simulink model "ModeSelectionRing"  (R2020a)
settings: Solver=FixedStepDiscrete  StartTime=0.0  StopTime=10.0  FixedStep=0.001  RelTol=1e-3  EnableMultiTasking=on
PostLoadFcn:
  | , if any(exist('dsrtsu_mdlpostloadfcn', 'file') ~= 0), dsrtsu_mdlpostloadfcn('Execute', bdroot); end,
InitFcn:
  | , if any(exist('rtifpga_mdlclblib', 'file') ~= 0), rtifpga_mdlclblib('Init', bdroot); end,
libraries: simulink x1
settings Model: DSRTSU_INTERNAL_RTI_VER=560  DSRTSU_INTERNAL_RTI_TYPE=rti1401  RTICANMMDATA=struct('GeneralSetupData',struct('modelroot','C:\Users\harjo\Git\MACFormulaGit\MicroAutobox\rings\Mode_Selection_Ring','generalsettings',struct('filesettings',struct('destfolder',struct('Name','RTICANMM_FILES','Check',1),'buildfolder',struct('Name','.','Check',1),'AbsDestfolder',struct('Name','C:\Users\harjo\Git\MACFormulaGit\MicroAutobox\rings\Mode_Selection_Ring\RTICANMM_FILES'),'AbsBuildfolder',struct('Name','C:\Users\harjo\Git\MACFormulaGit\MicroAutobox\rings\Mode_Selection_Ring'))),'options',struct('addpaths',1,'rmpaths',1,'addtrcexclusion',true,'cannavigator',struct('checkmonitoring',0),'show_usrtrc',0,'use_usrtrc',0),'advanced',struct('options',ones(1,100)),'MPSetup',{{}},'RTI',struct('Type','RTI1401','Ver','7.14','Date','02-May-2020'),'modelname','ModeSelectionRing','block','ModeSelectionRing'))  DSRTSU_INTERNAL_RTIFPGA=160  Creator=Harjot  LastModifiedBy=Harjot
settings DebuggingCC: SFUnexpectedBacktrackingDiag=warning  SFNoUnconditionalDefaultTransitionDiag=warning  SFExecutionAtInitializationDiag=none  ArithmeticOperatorsInVariantConditions=warning
settings HardwareCC: ProdBitPerPointer=32  ProdBitPerSizeT=32  ProdBitPerPtrDiffT=32  ProdLargestAtomicInteger=Integer  ProdEndianess=BigEndian  ProdWordSize=32  ProdHWDeviceType=Custom Processor->Custom  TargetIntDivRoundTo=Zero  TargetEndianess=BigEndian  TargetHWDeviceType=Custom Processor->Custom
settings SFSimCC: SimUseLocalCustomCode=off  MATLABDynamicMemAlloc=off  CustomCodeUndefinedFunction=UseInterfaceOnly
settings RTWCC: Description=dSPACE DS1401 Hardware Platform  SystemTargetFile=rti1401.tlc  MakeCommand=make_rti  TemplateMakefile=rti1401.tmf  RTWUseLocalCustomCode=off
settings CodeAppCC: StateflowObjectComments=on
settings STFCustomTargetCC: UtilityFuncGeneration=Shared location  ParMdlRefBuildCompliant=on  SystemTargetFile=rti1401.tlc
settings GRTTargetCC: TargetLangStandard=C89/C90 (ANSI)  UtilityFuncGeneration=Shared location  CompOptLevelCompliant=off  ConcurrentExecutionCompliant=off  CombineOutputUpdateFcns=off  MatFileLogging=off  CPPClassGenCompliant=off  UseToolchainInfoCompliant=off
settings ConfigComp: CovMetricSettings=dw  CovHtmlReporting=on  CovSaveCumulativeToWorkspaceVar=on  CovSaveSingleToWorkspaceVar=on  CovExternalEMLEnable=off

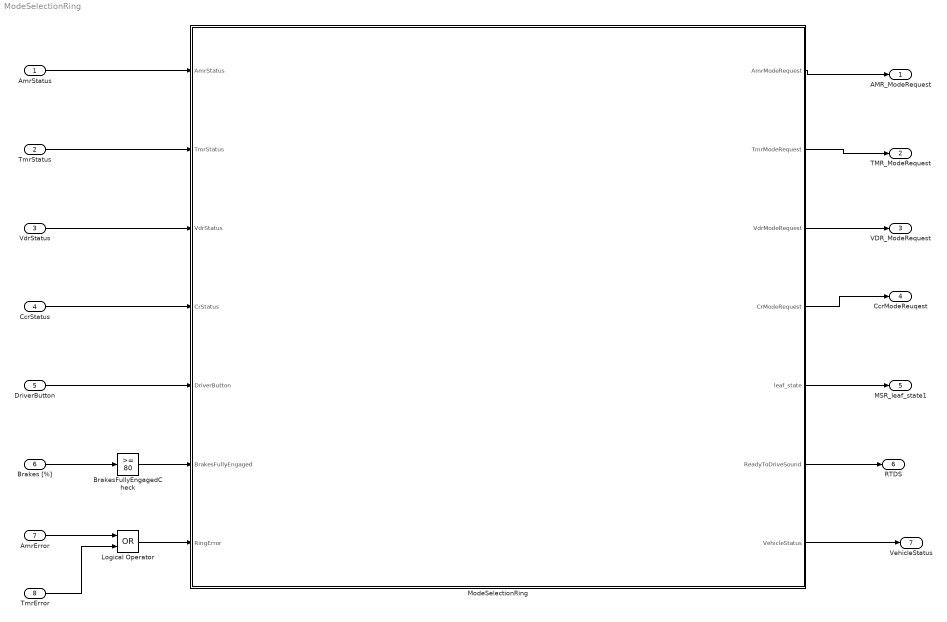
== system ModeSelectionRing ==
  AmrStatus : Inport
  TmrStatus : Inport  Port=2
  VdrStatus : Inport  Port=3
  CcrStatus : Inport  Port=4
  DriverButton : Inport  Port=5
  Brakes [%] : Inport  Port=6
  AmrError : Inport  Port=7
  TmrError : Inport  Port=8
  BrakesFullyEngagedCheck : simulink/Logic and Bit Operations/Compare To Constant  relop=>=  const=80  OutDataTypeStr=boolean
  Logical Operator : Logic  Operator=OR  AllPortsSameDT=off  OutDataTypeStr=boolean
  ModeSelectionRing : Stateflow chart  TreatAsAtomicUnit=on
  AMR_ModeRequest : Outport  VectorParamsAs1DForOutWhenUnconnected=off
  TMR_ModeRequest : Outport  Port=2  VectorParamsAs1DForOutWhenUnconnected=off
  VDR_ModeRequest : Outport  Port=3  VectorParamsAs1DForOutWhenUnconnected=off
  CcrModeReuqest : Outport  Port=4  VectorParamsAs1DForOutWhenUnconnected=off
  MSR_leaf_state1 : Outport  Port=5  VectorParamsAs1DForOutWhenUnconnected=off
  RTDS : Outport  Port=6  VectorParamsAs1DForOutWhenUnconnected=off
  VehicleStatus : Outport  Port=7  VectorParamsAs1DForOutWhenUnconnected=off
  wires:
  AmrStatus/1 -> ModeSelectionRing/1(AmrStatus)
  TmrStatus/1 -> ModeSelectionRing/2(TmrStatus)
  VdrStatus/1 -> ModeSelectionRing/3(VdrStatus)
  CcrStatus/1 -> ModeSelectionRing/4(CrStatus)
  DriverButton/1 -> ModeSelectionRing/5(DriverButton)
  ModeSelectionRing/1(AmrModeRequest) -> AMR_ModeRequest/1
  ModeSelectionRing/2(TmrModeRequest) -> TMR_ModeRequest/1
  ModeSelectionRing/3(VdrModeRequest) -> VDR_ModeRequest/1
  ModeSelectionRing/6(ReadyToDriveSound) -> RTDS/1
  ModeSelectionRing/5(leaf_state) -> MSR_leaf_state1/1
  ModeSelectionRing/4(CrModeRequest) -> CcrModeReuqest/1
  ModeSelectionRing/7(VehicleStatus) -> VehicleStatus/1
  Brakes [%]/1 -> BrakesFullyEngagedCheck/1
  BrakesFullyEngagedCheck/1 -> ModeSelectionRing/6(BrakesFullyEngaged)
  AmrError/1 -> Logical Operator/1
  TmrError/1 -> Logical Operator/2
  Logical Operator/1 -> ModeSelectionRing/7(RingError)

== stateflow chart ModeSelectionRing/ModeSelectionRing ==
  state OPERATION
    state STARTUP
      entry:
      VehicleStatus = VEHICLE_STATUS.LOCK;
      state HIGH_VOLTAGE
        state HIGH_VOLTAGE_STARTUP_FAIL
          entry:
        state ACCUMULATOR_HV_STARTUP
          state ACCUMULATOR_HV_REQUEST_STARTUP
            entry:
            AmrModeRequest = MSR_REQUEST.STARTUP_HV;
          state ACCUMULATOR_HV_STARTUP_FAIL
            entry:
            accumulatorHvStartupFail = true;
          state ACCUMULATOR_HV_STARTUP_PASS
            entry:
            accumulatorHvStartupPass = true;
          (default) -> OPERATION.STARTUP.HIGH_VOLTAGE.ACCUMULATOR_HV_STARTUP.ACCUMULATOR_HV_REQUEST_STARTUP
          OPERATION.STARTUP.HIGH_VOLTAGE.ACCUMULATOR_HV_STARTUP.ACCUMULATOR_HV_REQUEST_STARTUP -> OPERATION.STARTUP.HIGH_VOLTAGE.ACCUMULATOR_HV_STARTUP.ACCUMULATOR_HV_STARTUP_FAIL [order 2] : after(10,sec)
          OPERATION.STARTUP.HIGH_VOLTAGE.ACCUMULATOR_HV_STARTUP.ACCUMULATOR_HV_REQUEST_STARTUP -> OPERATION.STARTUP.HIGH_VOLTAGE.ACCUMULATOR_HV_STARTUP.ACCUMULATOR_HV_STARTUP_PASS [order 1] : [AmrStatus == RING_STATUS.STARTUP_COMPLETE_HV]
        state MOTORS_HV_STARTUP
          state MOTORS_HV_REQUEST_STARTUP
            entry:
            TmrModeRequest = MSR_REQUEST.STARTUP_HV;
          state MOTORS_HV_STARTUP_FAIL
            entry:
            motorHvStartupFail = true;
          state MOTORS_HV_STARTUP_PASS
            entry:
            motorHvStartupPass = true;
          (default) -> MOTORS_HV_REQUEST_STARTUP
          MOTORS_HV_REQUEST_STARTUP -> MOTORS_HV_STARTUP_FAIL [order 2] : after(10,sec)
          MOTORS_HV_REQUEST_STARTUP -> MOTORS_HV_STARTUP_PASS [order 1] : [TmrStatus == RING_STATUS.STARTUP_COMPLETE_HV]
        state VEHICLE_DYNAMICS_STARTUP
          state VEHICLE_DYANMICS_REQUEST_STARTUP
            entry:
            VdrModeRequest = MSR_REQUEST.STARTUP_HV;
          state VEHICLE_DYANMICS_STARTUP_FAIL
            entry:
            vehicleDynamicsStartupFail = true;
          state VEHICLE_DYANMICS_STARTUP_PASS
            entry:
            vehicleDynamicsStartupPass = true;
          (default) -> VEHICLE_DYANMICS_REQUEST_STARTUP
          VEHICLE_DYANMICS_REQUEST_STARTUP -> VEHICLE_DYANMICS_STARTUP_FAIL [order 2] : after(10,sec)
          VEHICLE_DYANMICS_REQUEST_STARTUP -> VEHICLE_DYANMICS_STARTUP_PASS [order 1] : [VdrStatus == RING_STATUS.STARTUP_COMPLETE_HV]
        (default) -> OPERATION.STARTUP.HIGH_VOLTAGE.ACCUMULATOR_HV_STARTUP
        OPERATION.STARTUP.HIGH_VOLTAGE.ACCUMULATOR_HV_STARTUP -> HIGH_VOLTAGE_STARTUP_FAIL [order 2] : [accumulatorHvStartupFail]
        OPERATION.STARTUP.HIGH_VOLTAGE.ACCUMULATOR_HV_STARTUP -> MOTORS_HV_STARTUP [order 1] : [accumulatorHvStartupPass]
        MOTORS_HV_STARTUP -> HIGH_VOLTAGE_STARTUP_FAIL [order 2] : [motorHvStartupFail]
        MOTORS_HV_STARTUP -> VEHICLE_DYNAMICS_STARTUP [order 1] : [motorHvStartupPass]
        VEHICLE_DYNAMICS_STARTUP -> HIGH_VOLTAGE_STARTUP_FAIL [order 2] : [vehicleDynamicsStartupFail]
      state LOW_VOLTAGE_STARTUP_FAIL
        entry:
      state COOLING_STARTUP
        state COOLING_REQUEST_STARTUP
          entry:
          CrModeRequest = MSR_REQUEST.STARTUP_LV;
        state COOLING_STARTUP_FAIL
          entry:
          coolingStartupFail = true;
        state COOLING_STARTUP_PASS
          entry:
          coolingStartupPass = true;
        (default) -> COOLING_REQUEST_STARTUP
        COOLING_REQUEST_STARTUP -> COOLING_STARTUP_FAIL [order 2] : after(10,sec)
        COOLING_REQUEST_STARTUP -> COOLING_STARTUP_PASS [order 1] : [CrStatus == RING_STATUS.STARTUP_COMPLETE_LV]
      state WAITING_FOR_RTD_AND_BRAKES1
        entry:
        internalShutdown = true;
      state MOTORS_LV_STARTUP
        state MOTORS_LV_REQUEST_STARTUP
          entry:
          TmrModeRequest = MSR_REQUEST.STARTUP_LV;
        state MOTORS_LV_STARTUP_FAIL
          entry:
          motorLvStartupFail = true;
        state MOTORS_LV_STARTUP_PASS
          entry:
          motorLvStartupPass = true;
        (default) -> MOTORS_LV_REQUEST_STARTUP
        MOTORS_LV_REQUEST_STARTUP -> MOTORS_LV_STARTUP_FAIL [order 2] : after(10,sec)
        MOTORS_LV_REQUEST_STARTUP -> MOTORS_LV_STARTUP_PASS [order 1] : [TmrStatus == RING_STATUS.STARTUP_COMPLETE_LV]
      state WAITING_FOR_RTD_AND_BRAKES
        entry:
        VehicleStatus = VEHICLE_STATUS.ACCESSORY;
      state ReadyToDriveSoundStart
        entry:
        ReadyToDriveSound = true;
        exit:
        ReadyToDriveSound = false;
      state ReadyToDriveSoundEnd
        entry:
        vehicleReady = true;
      (default) -> COOLING_STARTUP
      COOLING_STARTUP -> LOW_VOLTAGE_STARTUP_FAIL [order 2] : [coolingStartupFail]
      COOLING_STARTUP -> MOTORS_LV_STARTUP [order 1] : [coolingStartupPass]
      HIGH_VOLTAGE -> WAITING_FOR_RTD_AND_BRAKES1 : [~BrakesFullyEngaged]
      MOTORS_LV_STARTUP -> LOW_VOLTAGE_STARTUP_FAIL [order 1] : [motorLvStartupFail]
      MOTORS_LV_STARTUP -> WAITING_FOR_RTD_AND_BRAKES [order 2] : [motorLvStartupPass]
      WAITING_FOR_RTD_AND_BRAKES -> HIGH_VOLTAGE : [DriverButton == DRIVER_BUTTON.ON && BrakesFullyEngaged]
      VEHICLE_DYNAMICS_STARTUP -> ReadyToDriveSoundStart [order 1] : [vehicleDynamicsStartupPass]
      ReadyToDriveSoundStart -> ReadyToDriveSoundEnd : [after(3.5,sec) ]
    state SYSTEM_MODE_SELECTION
      entry:
      VehicleStatus = VEHICLE_STATUS.ON;
      state SAFE
      state NORMAL
        during:
        AmrModeRequest = MSR_REQUEST.RUNNING;
        TmrModeRequest = MSR_REQUEST.RUNNING;
        VdrModeRequest = MSR_REQUEST.RUNNING;
        CrModeRequest = MSR_REQUEST.RUNNING;
      state LOW_POWER
      state SHUTDOWN_BEGIN
      state Functions [group] [commented out]
      SAFE -> SHUTDOWN_BEGIN : E_Shutdown
      LOW_POWER -> SAFE [order 2] : E_Safe
      NORMAL -> SAFE [order 1] : E_Safe
      (default) -> NORMAL
      NORMAL -> LOW_POWER [order 2] : E_LowPower
      NORMAL -> SHUTDOWN_BEGIN [order 3] : E_Shutdown
      LOW_POWER -> SHUTDOWN_BEGIN [order 1] : E_Shutdown
    (default) -> STARTUP
    STARTUP -> SYSTEM_MODE_SELECTION : [vehicleReady]
  state SHUTDOWN
    state SHUTDOWN_FAIL
    state VEHICLE_DYNAMICS_SHUTDOWN
      state VEHICLE_DYANMICS_REQUEST_SHUTDOWN
        entry:
        VdrModeRequest = MSR_REQUEST.SHUTDOWN_HV;
      state VEHICLE_DYANMICS_SHUTDOWN_FAIL
        entry:
        vehicleDynamicsShutdownFail = true;
      state VEHICLE_DYANMICS_SHUTDOWN_PASS
        entry:
        vehicleDynamicsShutdownPass = true;
      (default) -> VEHICLE_DYANMICS_REQUEST_SHUTDOWN
      VEHICLE_DYANMICS_REQUEST_SHUTDOWN -> VEHICLE_DYANMICS_SHUTDOWN_FAIL [order 2] : after(3,sec)
      VEHICLE_DYANMICS_REQUEST_SHUTDOWN -> VEHICLE_DYANMICS_SHUTDOWN_PASS [order 1] : [VdrStatus == RING_STATUS.SHUTDOWN_COMPLETE_HV]
    state TRACTIVE_SYSTEM_SHUTDOWN
      state MOTORS_HV_SHUTDOWN [parallel]
        settings: executionOrder=1
        state MOTORS_HV_REQUEST_SHUTDOWN
          entry:
          TmrModeRequest = MSR_REQUEST.SHUTDOWN_HV;
        state MOTORS_HV_SHUTDOWN_FAIL
          entry:
          motorHvShutdownFail = true;
        state MOTORS_HV_SHUTDOWN_PASS
          entry:
          motorHvShutdownPass = true;
        (default) -> MOTORS_HV_REQUEST_SHUTDOWN
        MOTORS_HV_REQUEST_SHUTDOWN -> MOTORS_HV_SHUTDOWN_FAIL [order 2] : after(3,sec)
        MOTORS_HV_REQUEST_SHUTDOWN -> MOTORS_HV_SHUTDOWN_PASS [order 1] : [TmrStatus == RING_STATUS.SHUTDOWN_COMPLETE_HV]
      state ACCUMULATOR_HV_STARTUP [parallel]
        settings: executionOrder=2
        state ACCUMULATOR_HV_REQUEST_STARTUP
          entry:
          AmrModeRequest = MSR_REQUEST.SHUTDOWN_HV;
        state ACCUMULATOR_HV_STARTUP_FAIL
          entry:
          accumulatorHvShutdownFail = true;
        state ACCUMULATOR_HV_STARTUP_PASS
          entry:
          accumulatorHvShutdownPass = true;
        (default) -> SHUTDOWN.TRACTIVE_SYSTEM_SHUTDOWN.ACCUMULATOR_HV_STARTUP.ACCUMULATOR_HV_REQUEST_STARTUP
        SHUTDOWN.TRACTIVE_SYSTEM_SHUTDOWN.ACCUMULATOR_HV_STARTUP.ACCUMULATOR_HV_REQUEST_STARTUP -> SHUTDOWN.TRACTIVE_SYSTEM_SHUTDOWN.ACCUMULATOR_HV_STARTUP.ACCUMULATOR_HV_STARTUP_FAIL [order 2] : after(3,sec)
        SHUTDOWN.TRACTIVE_SYSTEM_SHUTDOWN.ACCUMULATOR_HV_STARTUP.ACCUMULATOR_HV_REQUEST_STARTUP -> SHUTDOWN.TRACTIVE_SYSTEM_SHUTDOWN.ACCUMULATOR_HV_STARTUP.ACCUMULATOR_HV_STARTUP_PASS [order 1] : [AmrStatus == RING_STATUS.SHUTDOWN_COMPLETE_HV]
    state COOLING_SHUTDOWN
      state COOLING_REQUEST_SHUTDOWN
        entry:
        CrModeRequest = MSR_REQUEST.SHUTDOWN_LV;
      state COOLING_SHUTDOWN_FAIL
        entry:
        coolingShutdownFail = true;
      state COOLING_SHUTDOWN_PASS
        entry:
        coolingShutdownPass = true;
      (default) -> COOLING_REQUEST_SHUTDOWN
      COOLING_REQUEST_SHUTDOWN -> COOLING_SHUTDOWN_FAIL [order 2] : after(10,sec)
      COOLING_REQUEST_SHUTDOWN -> COOLING_SHUTDOWN_PASS [order 1] : [CrStatus == RING_STATUS.SHUTDOWN_COMPLETE_LV]
    state ShutdownComplete
      entry:
      VehicleStatus = VEHICLE_STATUS.SHUTDOWN;
    (default) -> VEHICLE_DYNAMICS_SHUTDOWN
    VEHICLE_DYNAMICS_SHUTDOWN -> SHUTDOWN_FAIL [order 2] : [vehicleDynamicsShutdownFail]
    VEHICLE_DYNAMICS_SHUTDOWN -> TRACTIVE_SYSTEM_SHUTDOWN [order 1] : [vehicleDynamicsShutdownPass]
    TRACTIVE_SYSTEM_SHUTDOWN -> SHUTDOWN_FAIL [order 2] : [motorHvShutdownFail &&...
        | accumulatorHvShutdownFail]
    TRACTIVE_SYSTEM_SHUTDOWN -> COOLING_SHUTDOWN [order 1] : [motorHvShutdownPass && accumulatorHvShutdownPass]
    COOLING_SHUTDOWN -> SHUTDOWN_FAIL [order 2] : [coolingShutdownFail]
    COOLING_SHUTDOWN -> ShutdownComplete [order 1] : [coolingShutdownPass]
  (default) -> OPERATION
  OPERATION -> SHUTDOWN : [DriverButton == DRIVER_BUTTON.SHUTDOWN ||...
      |  internalShutdown || RingError]
  data: AmrStatus input Enum: RING_STATUS; TmrStatus input Enum: RING_STATUS; VdrStatus input Enum: RING_STATUS; CrStatus input Enum: RING_STATUS; AmrModeRequest output Enum: MSR_REQUEST; TmrModeRequest output Enum: MSR_REQUEST; VdrModeRequest output Enum: MSR_REQUEST; CrModeRequest output Enum: MSR_REQUEST; DriverButton input Enum: DRIVER_BUTTON; internalShutdown local boolean =false; leaf_state output Enum: MSR_States; BrakesFullyEngaged input boolean; ReadyToDriveSound output; motorLvStartupFail local boolean =false; motorLvStartupPass local boolean =false; vehicleDynamicsStartupPass local boolean =false; vehicleDynamicsStartupFail local boolean =false; coolingStartupFail local boolean =false; coolingStartupPass local boolean =false; accumulatorLvStartupFail local boolean =false; accumulatorLvStartupPass local boolean =false; accumulatorHvStartupFail local boolean =false; motorHvStartupFail local boolean =false; motorHvStartupPass local boolean =false; vehicleReady local boolean =false; accumulatorHvStartupPass local boolean =false; motorHvShutdownPass local boolean =false; motorHvShutdownFail local boolean =false; coolingShutdownPass local boolean =false; coolingShutdownFail local boolean =false; accumulatorHvShutdownFail local boolean =false; vehicleDynamicsShutdownFail local boolean =false; vehicleDynamicsShutdownPass local boolean =false; accumulatorHvShutdownPass local boolean =false; VehicleStatus output Enum: VEHICLE_STATUS; RingError input boolean
  events: E_LowPower local FUNCTION_CALL_EVENT; E_Shutdown local FUNCTION_CALL_EVENT; E_Safe local FUNCTION_CALL_EVENT
  function CHECKING_CONDITIONS:
    | function CHECKING_CONDITIONS
    | cond1 = false;
    | cond2 = false;
    | cond3 = false;
    | cond4 = false;
    | cond5 = false;
    | cond6 = false;
    | cond7 = false;
    | cond8 = false;
    | cond9 = false;
    | cond10 = false;
    | cond11 = false;
    | cond12 = false;
    | cond13 = false;
    | cond14 = false;
    | cond15 = false;
    | cond16 = false;
    | cond17 = false;
    | cond18 = false;
    | cond19 = false;
    | cond20 = false;
    | cond21 = false;
    | if (cond1 || cond2)
    |     %cond1 = BMR.State.Startup_LowEnergy
    |     %cond2 = BMR.State.Running_LowEnergy
    |     send(E_LowPower);
    | elseif (cond3 || cond4 || cond5 || cond6)
    |     %cond3 = CCR.MotorTempSensorFail
    |     %cond4 = CCR.FluidTempSensorFail
    |     %cond5 = CCR.FanRPMSensorFail
    |     %cond6 = CCR.CmpFail
    |     send(E_Safe);
    | elseif (cond7 || cond8 || cond9 || cond10 || cond11 || cond12 || ...
    |         cond13 || cond14 || cond15 || cond16 || cond17 || cond18 ...
    |         || cond19 || cond20 || cond21)
    |     %cond7 = VDR_Status.APPS_Fail
    |     %cond8 = VDR_Status.BSE_Fail
    |     %cond9 = VDR_Status.Motor_Fail  (vector of size 1x4 for each motor)
    |     %cond10 = VDR_Status.Over_Torque
    |     %cond11 = VDR_Status.CAN_Fault
    |     %cond12 = TMR_Status.Over_Torque
    |     %cond13 = TMR_Status.CAN_Fault
    |     %cond14 = TMR_Status.Under_Torque
    |     %cond15 = TMR_Status.AMK_Sensor_Fail
    |     %cond16 = TMR_Status.Startup_Fail
    |     %cond17 = TMR_Status.Motor_Fail  (vector of size 1x4 for each motor)
    |     %cond18 = AMR.State.Startup_Fail
    |     %cond19 = AMR.State.Running_GenFail
    |     %cond20 = AMR.State.Cell_OutofLmt
    |     %cond21 = AMR.State.Sensor_Fail
    |     send(E_Shutdown);
    | end
  function SHUTDOWN_MOTORS:
    | function SHUTDOWN_MOTORS
